simulink model "SIL_PIL_torque_controller_model"  (R2023b)
settings: Solver=FixedStepAuto  StartTime=0.0  StopTime=10.0  RelTol=1e-3  EnableMultiTasking=on
undefined symbols (not defined in the file): DiscIntNeverNeededParam, K, Kp, Ti, Ts
settings Model: ExtModeTrigDuration=10  Creator=kiraa  LastModifiedBy=kiraa
settings OptimizationCC: EnhancedBackFolding=on  PassReuseOutputArgsAs=Individual arguments  ZeroExternalMemoryAtStartup=off  ZeroInternalMemoryAtStartup=off  MaxStackSize=64  OptimizeBlockOrder=speed  DifferentSizesBufferReuse=on  OptimizationCustomize=off  EfficientTunableParamExpr=on
settings DebuggingCC: ParameterTunabilityLossMsg=error
settings HardwareCC: ProdBitPerPointer=32  ProdBitPerSizeT=32  ProdBitPerPtrDiffT=32  ProdLargestAtomicInteger=Long  ProdLargestAtomicFloat=Double  ProdWordSize=32  ProdLongLongMode=on  ProdHWDeviceType=ARM Compatible->ARM Cortex
settings SFSimCC: MATLABDynamicMemAlloc=off
settings RTWCC: Description=Embedded Coder  SystemTargetFile=ert.tlc  HardwareBoard=STM32 Nucleo F401RE  TemplateMakefile=ert_default_tmf  Toolchain=GNU Tools for ARM Embedded Processors
settings CodeAppCC: ForceParamTrailComments=on  IgnoreCustomStorageClasses=off  OperatorAnnotations=on  SimulinkDataObjDesc=on  SFDataObjDesc=on  InsertBlockDesc=on
settings ERTTargetCC: ExtModeTransport=3  ExtModeStaticAlloc=on  ExtModeStaticAllocSize=2000  ExtModeMexFile=ext_xcp  ExtModeIntrfLevel=Level2 - Open

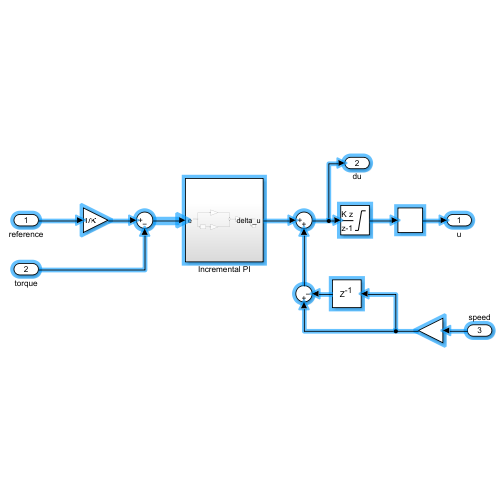
[thumbnail: Simulink's stored preview of the top-level diagram]
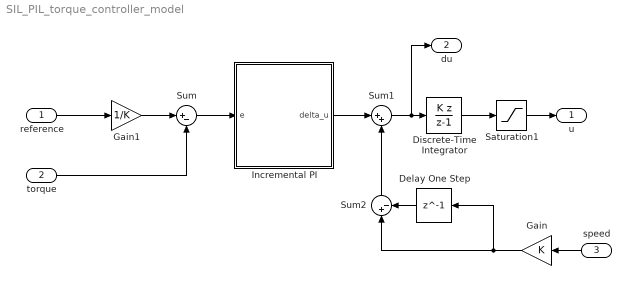
== system SIL_PIL_torque_controller_model ==
  reference : Inport
  torque : Inport  Port=2
  speed : Inport  Port=3
  Delay One Step : Delay  DelayLength=1
  Discrete-Time Integrator : DiscreteIntegrator  IntegratorMethod=Accumulation: Backward Euler  SampleTime=-1  LimitOutput=on  UpperSaturationLimit=12  LowerSaturationLimit=-12  ICPrevOutput=DiscIntNeverNeededParam  ICPrevScaledInput=DiscIntNeverNeededParam
  Gain : Gain  Gain=K
  Gain1 : Gain  Gain=1/K
  Incremental PI : Subsystem
  Saturation1 : Saturate  UpperLimit=12  LowerLimit=-12
  Sum : Sum  Inputs=|+-
  Sum1 : Sum  Inputs=|++
  Sum2 : Sum  Inputs=|+-
  u : Outport
  du : Outport  Port=2
  wires:
  Gain/1 -> Sum2/1, Delay One Step/1
  Sum2/1 -> Sum1/2
  Incremental PI/1(delta_u) -> Sum1/1
  Saturation1/1 -> u/1
  reference/1 -> Gain1/1
  Discrete-Time Integrator/1 -> Saturation1/1
  Sum1/1 -> du/1, Discrete-Time Integrator/1
  torque/1 -> Sum/2
  speed/1 -> Gain/1
  Gain1/1 -> Sum/1
  Delay One Step/1 -> Sum2/2
  Sum/1 -> Incremental PI/1(e)

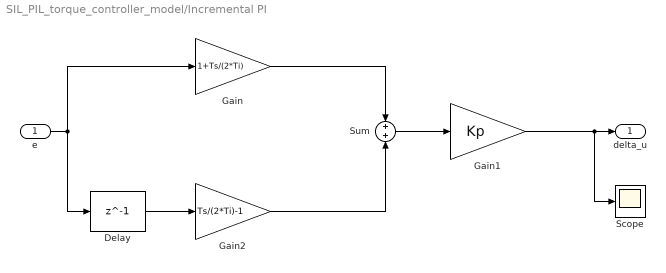
== system SIL_PIL_torque_controller_model/Incremental PI ==
  e : Inport  SampleTime=Ts
  Delay : Delay  DelayLength=1  InitialCondition=0  UseCircularBuffer=on
  Gain : Gain  Gain=1+Ts/(2*Ti)
  Gain1 : Gain  Gain=Kp
  Gain2 : Gain  Gain=Ts/(2*Ti)-1
  Scope : Scope
  Sum : Sum  Inputs=+|+
  delta_u : Outport  SampleTime=Ts
  wires:
  e/1 -> Delay/1, Gain/1
  Delay/1 -> Gain2/1
  Gain/1 -> Sum/1
  Sum/1 -> Gain1/1
  Gain1/1 -> Scope/1, delta_u/1
  Gain2/1 -> Sum/2
